simulink model "Prova_SITL_GPS_cost"  (R2020b)
settings: Solver=VariableStepAuto  StartTime=0.0  StopTime=10.0  RelTol=1e-3
settings Model: Creator=SUSANNA  LastModifiedBy=SUSANNA
settings DebuggingCC: UnconnectedInputMsg=none  UnconnectedOutputMsg=none  UnconnectedLineMsg=none  SFMachineParentedDataDiag=error
settings ModelReferenceCC: EnableRefExpFcnMdlSchedulingChecks=off

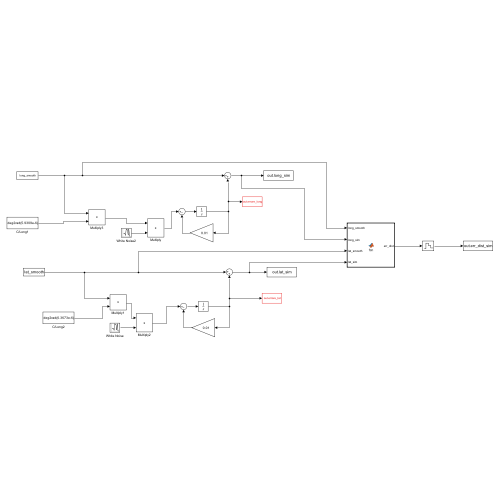
[thumbnail: Simulink's stored preview of the top-level diagram]
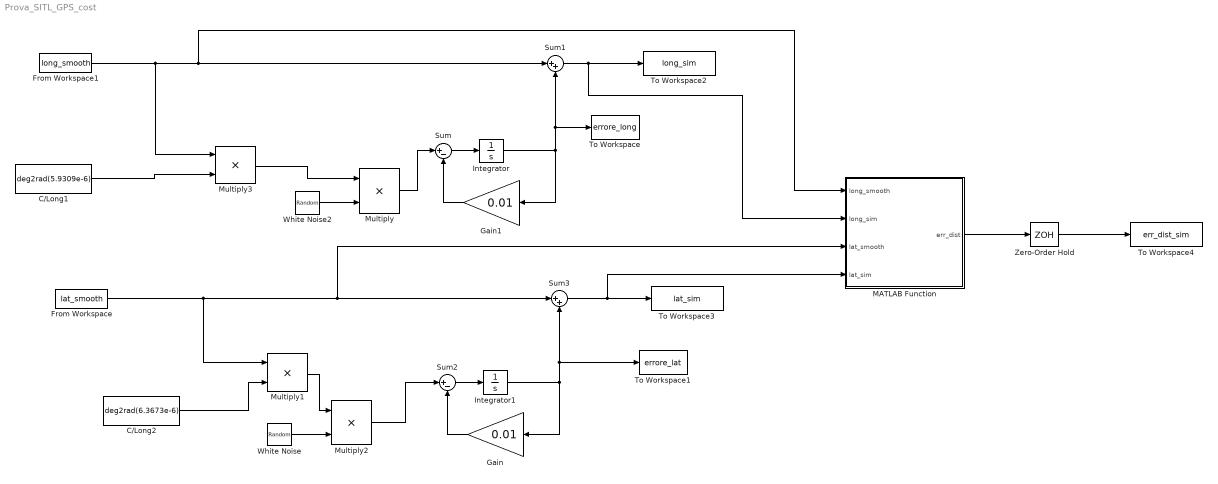
== system Prova_SITL_GPS_cost ==
  C/Long1 : Constant  Value=deg2rad(5.9309e-6)
  C/Long2 : Constant  Value=deg2rad(6.3673e-6)
  From Workspace : FromWorkspace  VariableName=lat_smooth
  From Workspace1 : FromWorkspace  VariableName=long_smooth
  Gain : Gain  Gain=0.01  SaturateOnIntegerOverflow=on  OutDataTypeStr=Inherit: Same as input  ParamDataTypeStr=Inherit: Same as input
  Gain1 : Gain  Gain=0.01  SaturateOnIntegerOverflow=on  OutDataTypeStr=Inherit: Same as input  ParamDataTypeStr=Inherit: Same as input
  Integrator : Integrator
  Integrator1 : Integrator
  MATLAB Function : MATLAB Function  TreatAsAtomicUnit=on
  Multiply{,1..3} (4 alike) : Product
  Sum : Sum  Inputs=|+-  InputSameDT=on  SaturateOnIntegerOverflow=on  OutDataTypeStr=Inherit: Same as first input
  Sum1 : Sum  Inputs=|++  InputSameDT=on  SaturateOnIntegerOverflow=on  OutDataTypeStr=Inherit: Same as first input
  Sum2 : Sum  Inputs=|+-  InputSameDT=on  SaturateOnIntegerOverflow=on  OutDataTypeStr=Inherit: Same as first input
  Sum3 : Sum  Inputs=|++  InputSameDT=on  SaturateOnIntegerOverflow=on  OutDataTypeStr=Inherit: Same as first input
  To Workspace : ToWorkspace  VariableName=errore_long  SampleTime=-1
      settings: Save2DSignal=2-D array (concatenate along first dimension)
  To Workspace1 : ToWorkspace  VariableName=errore_lat  SampleTime=-1
      settings: Save2DSignal=2-D array (concatenate along first dimension)
  To Workspace2 : ToWorkspace  VariableName=long_sim  SampleTime=-1
      settings: Save2DSignal=2-D array (concatenate along first dimension)
  To Workspace3 : ToWorkspace  VariableName=lat_sim  SampleTime=-1
      settings: Save2DSignal=2-D array (concatenate along first dimension)
  To Workspace4 : ToWorkspace  VariableName=err_dist_sim  SampleTime=-1
      settings: Save2DSignal=2-D array (concatenate along first dimension)
  White Noise : RandomNumber  Seed=randi([0 2000],1,1)  SampleTime=0.1
  White Noise2 : RandomNumber  Seed=randi([0 2000],1,1)  SampleTime=0.1
  Zero-Order Hold : ZeroOrderHold  SampleTime=0.02
  wires:
  C/Long2/1 -> Multiply1/2
  Multiply2/1 -> Sum2/1
  Gain1/1 -> Sum/2
  Sum3/1 -> MATLAB Function/4(lat_sim), To Workspace3/1
  Zero-Order Hold/1 -> To Workspace4/1
  Gain/1 -> Sum2/2
  C/Long1/1 -> Multiply3/2
  Multiply/1 -> Sum/1
  White Noise2/1 -> Multiply/2
  White Noise/1 -> Multiply2/2
  Sum2/1 -> Integrator1/1
  Integrator/1 -> Sum1/2, To Workspace/1, Gain1/1
  Integrator1/1 -> Gain/1, Sum3/2, To Workspace1/1
  Sum/1 -> Integrator/1
  MATLAB Function/1(err_dist) -> Zero-Order Hold/1
  Sum1/1 -> MATLAB Function/2(long_sim), To Workspace2/1
  From Workspace1/1 -> Multiply3/1, MATLAB Function/1(long_smooth), Sum1/1
  Multiply3/1 -> Multiply/1
  From Workspace/1 -> Multiply1/1, MATLAB Function/3(lat_smooth), Sum3/1
  Multiply1/1 -> Multiply2/1

== matlab function Prova_SITL_GPS_cost/MATLAB Function ==
  data: long_smooth input; long_sim input; lat_smooth input; err_dist output; lat_sim input
function err_dist = fcn(long_smooth,long_sim,lat_smooth,lat_sim )

r=6371*10^3; %raggio terra in m


err_dist = 2*r*asin(sqrt(sin((lat_smooth-lat_sim)/2)^2+cos(lat_sim)*cos(lat_smooth)*sin((long_smooth-long_sim)/2)^2 ));
